simulink model "Regelstrecke"  (Simulink 9.1)
settings: Solver=ode23  StartTime=0.0  StopTime=10  FixedStep=0.015  RelTol=1e-3  EnableMultiTasking=on
PreLoadFcn:
  | pruefzylinder
  | pruefling
undefined symbols (not defined in the file): b1, c_oe, c_p, m_g
settings Model: Creator=yjl_9  LastModifiedBy=Emily
settings DataIOCC: LimitDataPoints=on
settings DebuggingCC: SolverPrmCheckMsg=warning
settings GRTTargetCC: GeneratePreprocessorConditionals=Disable all  CombineOutputUpdateFcns=on  GRTInterface=off

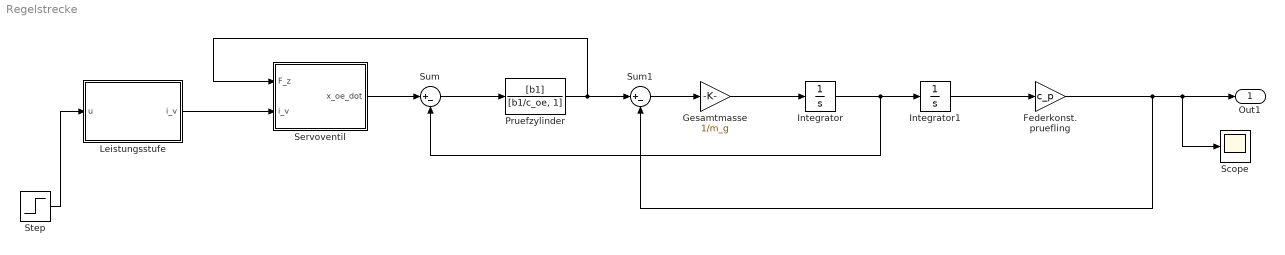
== system Regelstrecke ==
  Federkonst. pruefling : Gain  Gain=c_p
  Gesamtmasse : Gain  Gain=1/m_g
  Integrator : Integrator
  Integrator1 : Integrator
  "Leistungsstufe " : MATLAB Function  TreatAsAtomicUnit=on
  Pruefzylinder : TransferFcn  Numerator=[b1]  Denominator=[b1/c_oe, 1]
  Scope : Scope
  "Servoventil " : MATLAB Function  TreatAsAtomicUnit=on
  Step : Step  SampleTime=0
  Sum : Sum  Inputs=|+-
  Sum1 : Sum  Inputs=|+-
  Out1 : Outport
  wires:
  "Leistungsstufe "/1(i_v) -> "Servoventil "/2(i_v)
  "Servoventil "/1(x_oe_dot) -> Sum/1
  Sum/1 -> Pruefzylinder/1
  Pruefzylinder/1 -> "Servoventil "/1(F_z), Sum1/1
  Sum1/1 -> Gesamtmasse/1
  Gesamtmasse/1 -> Integrator/1
  Integrator1/1 -> Federkonst. pruefling/1
  Integrator/1 -> Sum/2, Integrator1/1
  Federkonst. pruefling/1 -> Sum1/2, Scope/1, Out1/1
  Step/1 -> "Leistungsstufe "/1(u)

== matlab function Servoventil  ==
  data: F_z input double; i_v input double; x_oe_dot output double
function x_oe_dot = servoventil(F_z,i_v)
%#codegen
K_sv = 0.796; % [m/As]
F_N = 63000; % [N]
A = 1-(F_z/F_N)*sign(i_v);

if A > 0
    x_oe_dot = i_v*K_sv*sqrt(A);
else 
    x_oe_dot = 0;
end

== matlab function Leistungsstufe  ==
  data: u input double; i_v output double
function i_v  = leistungsstufe(u)
%codegen
i_max = 1; % [A]
K_L = 1; % [A/V]
    if u > 1
        i_v = i_max;
    elseif u < -1
        i_v = -i_max;
    else 
        i_v = K_L*u;
    end
